simulink model "COMPONENT_MDL_Lag_QUAD_and_PEND_with_spin_rotors"  (R2021b)
(part 5 of 10)

    mt33 = [et183+et184+et185+et186+et187+et188+et189+et190+et191+et192+et193+et194+et195+et196+et197+et198+et199+et200+et201+et202+et203+et204+et205+et206+et207+et208+et209+et210+et211+et212+et213+et214+et215+et216+et217+et218+et219+et220+et221+et222+et223+et224,et149+et150+et151+et152+et153+et154+et155+et156+et157+et158+et159+et160+et161+et162+et163+et164+et165+et166+et167+et168+et169+et170+et171+et172+et173+et174+et175+et176+et177+et178+et179+et180+et181+et182,et124+et125+et126+et127+et128+et129+et130+et131+et132+et133+et134+et135+et136+et137+et138+et139+et140+et141+et142+et143+et144+et145+et146+et147+et148,et120+et121+et122+et123,et116+et117+et118+et119,0.0,et96+et97+et98+et99+et100+et101+et102+et103+et104+et105+et106+et107+et108+et109+et110+et111+et112+et113+et114+et115,et77+et78+et79+et80+et81+et82+et83+et84+et85+et86+et87+et88+et89+et90+et91+et92+et93+et94+et95,et59+et60+et61+et62+et63+et64+et65+et66+et67+et68+et69+et70+et71+et72+et73+et74+et75+et76];
    mt34 = [et272+et273+et274+et275+et276+et277+et278+et279+et280+et281+et282+et283+et284+et285+et286+et287+et288+et289+et290+et291+et292+et293+et294+et295+et296+et297+et298+et299,et260+et261+et262+et263+et264+et265+et266+et267+et268+et269+et270+et271,et250+et251+et252+et253+et254+et255+et256+et257+et258+et259,cos(THE_Phi).*(et248+et249).*(-1.0./2.0),sin(THE_Phi).*(et246+et247).*(-1.0./2.0),et244+et245,et237+et238+et239+et240+et241+et242+et243,et231+et232+et233+et234+et235+et236,et225+et226+et227+et228+et229+et230,et321+et322+et323+et324+et325+et326+et327+et328+et329+et330+et331,et313+et314+et315+et316+et317+et318+et319+et320,et310+et311+et312,et308+et309,et306+et307];
    mt35 = [cos(THE_Theta).*(THE_Psi_D.*Tv_Z_pend.*m_pend.*cos(THE_Psi).*2.0+THE_Psi_D.*cg_to_mot_H.*mprop.*cos(THE_Psi).*8.0+Lz_pend.*THE_Psi_D.*m_pend.*cos(THE_Psi).*cos(THE_Psi_pend).*cos(THE_Theta_pend)+Lz_pend.*THE_Psi_pend_D.*m_pend.*cos(THE_Psi).*cos(THE_Phi_pend).*cos(THE_Psi_pend).*2.0-Lz_pend.*THE_Psi_D.*m_pend.*cos(THE_Phi_pend).*sin(THE_Psi).*sin(THE_Psi_pend)-Lz_pend.*THE_Phi_pend_D.*m_pend.*cos(THE_Psi).*sin(THE_Phi_pend).*sin(THE_Psi_pend).*2.0-Lz_pend.*THE_Psi_pend_D.*m_pend.*cos(THE_Theta_pend).*sin(THE_Psi).*sin(THE_Psi_pend).*2.0-Lz_pend.*THE_Theta_pend_D.*m_pend.*cos(THE_Psi_pend).*sin(THE_Psi).*sin(THE_Theta_pend).*2.0-Lz_pend.*THE_Phi_pend_D.*m_pend.*cos(THE_Psi).*cos(THE_Phi_pend).*cos(THE_Psi_pend).*sin(THE_Theta_pend).*2.0-Lz_pend.*THE_Theta_pend_D.*m_pend.*cos(THE_Psi).*cos(THE_Psi_pend).*cos(THE_Theta_pend).*sin(THE_Phi_pend).*2.0+Lz_pend.*THE_Psi_D.*m_pend.*cos(THE_Psi_pend).*sin(THE_Psi).*sin(THE_Phi_pend).*sin(THE_Theta_pend)+Lz_pend.*THE_Psi_pend_D.*m_pend.*cos(THE_Psi).*sin(THE_Phi_pend).*sin(THE_Psi_pend).*sin(THE_Theta_pend).*2.0).*(-1.0./2.0),(m_pend.*(et304+et305))./1.2e+1,et302+et303,m_pend.*(et300+et301).*(-1.0./1.2e+1),0.0,0.0,0.0,0.0,0.0,0.0,0.0,0.0,0.0,0.0,0.0,0.0,0.0,0.0,0.0,0.0,0.0,0.0,0.0,0.0,0.0,0.0,0.0,0.0,0.0,0.0,0.0,et342+et343+et344+et345+et346];
    mt36 = [et339+et340+et341,et337+et338,et335.*et336,et332.*et333.*et334,(Lz_pend.*m_pend.*(THE_Phi_pend_D.*sin(THE_Theta).*sin(THE_Phi_pend).*sin(THE_Psi_pend)-THE_Psi_pend_D.*cos(THE_Phi_pend).*cos(THE_Psi_pend).*sin(THE_Theta).*2.0+THE_Phi_pend_D.*cos(THE_Theta).*cos(THE_Phi_pend).*sin(THE_Psi).*sin(THE_Psi_pend)+THE_Psi_pend_D.*cos(THE_Theta).*cos(THE_Psi_pend).*sin(THE_Psi).*sin(THE_Phi_pend).*2.0+THE_Phi_pend_D.*cos(THE_Phi_pend).*cos(THE_Psi_pend).*sin(THE_Theta).*sin(THE_Theta_pend)+THE_Theta_pend_D.*cos(THE_Psi_pend).*cos(THE_Theta_pend).*sin(THE_Theta).*sin(THE_Phi_pend).*2.0-THE_Psi_pend_D.*sin(THE_Theta).*sin(THE_Phi_pend).*sin(THE_Psi_pend).*sin(THE_Theta_pend).*2.0+THE_Theta_pend_D.*cos(THE_Theta).*cos(THE_Phi_pend).*cos(THE_Psi_pend).*cos(THE_Theta_pend).*sin(THE_Psi).*2.0-THE_Phi_pend_D.*cos(THE_Theta).*cos(THE_Psi_pend).*sin(THE_Psi).*sin(THE_Phi_pend).*sin(THE_Theta_pend)-THE_Psi_pend_D.*cos(THE_Theta).*cos(THE_Phi_pend).*sin(THE_Psi).*sin(THE_Psi_pend).*sin(THE_Theta_pend).*2.0))./2.0];
    mt37 = [m_pend.*cos(THE_Theta_pend).*(Lx_pend.^2.*THE_Theta_pend_D.*sin(THE_Theta_pend)-Ly_pend.^2.*THE_Theta_pend_D.*sin(THE_Theta_pend)+Ly_pend.^2.*THE_Theta_pend_D.*cos(THE_Psi_pend).^2.*sin(THE_Theta_pend)-Lz_pend.^2.*THE_Theta_pend_D.*cos(THE_Psi_pend).^2.*sin(THE_Theta_pend).*4.0+Ly_pend.^2.*THE_Psi_pend_D.*cos(THE_Psi_pend).*cos(THE_Theta_pend).*sin(THE_Psi_pend)-Lz_pend.^2.*THE_Psi_pend_D.*cos(THE_Psi_pend).*cos(THE_Theta_pend).*sin(THE_Psi_pend).*4.0).*(-1.0./6.0),(m_pend.*cos(THE_Theta_pend).*(Ly_pend.^2.*THE_Psi_pend_D.*2.0+Lx_pend.^2.*THE_Phi_pend_D.*sin(THE_Theta_pend)-Ly_pend.^2.*THE_Phi_pend_D.*sin(THE_Theta_pend)-Ly_pend.^2.*THE_Psi_pend_D.*cos(THE_Psi_pend).^2.*2.0+Lz_pend.^2.*THE_Psi_pend_D.*cos(THE_Psi_pend).^2.*8.0+Ly_pend.^2.*THE_Phi_pend_D.*cos(THE_Psi_pend).^2.*sin(THE_Theta_pend)-Lz_pend.^2.*THE_Phi_pend_D.*cos(THE_Psi_pend).^2.*sin(THE_Theta_pend).*4.0))./1.2e+1];
    mt38 = [m_pend.*cos(THE_Theta_pend).*(Ly_pend.^2.*THE_Theta_pend_D.*2.0-Ly_pend.^2.*THE_Theta_pend_D.*cos(THE_Psi_pend).^2.*2.0+Lz_pend.^2.*THE_Theta_pend_D.*cos(THE_Psi_pend).^2.*8.0-Ly_pend.^2.*THE_Phi_pend_D.*cos(THE_Psi_pend).*cos(THE_Theta_pend).*sin(THE_Psi_pend)+Lz_pend.^2.*THE_Phi_pend_D.*cos(THE_Psi_pend).*cos(THE_Theta_pend).*sin(THE_Psi_pend).*4.0).*(-1.0./1.2e+1),et349+et350+et351,et347+et348];
    mt39 = [Lz_pend.^2.*THE_Psi_pend_D.*m_pend.*cos(THE_Phi_pend).*sin(THE_Theta_pend).*(-2.0./3.0)-(Ly_pend.^2.*THE_Psi_pend_D.*m_pend.*cos(THE_Psi_pend).*sin(THE_Phi_pend).*sin(THE_Psi_pend))./6.0+Lz_pend.^2.*THE_Psi_pend_D.*m_pend.*cos(THE_Psi_pend).*sin(THE_Phi_pend).*sin(THE_Psi_pend).*(2.0./3.0)-(Ly_pend.^2.*THE_Psi_pend_D.*m_pend.*cos(THE_Phi_pend).*cos(THE_Psi_pend).^2.*sin(THE_Theta_pend))./6.0+Lz_pend.^2.*THE_Psi_pend_D.*m_pend.*cos(THE_Phi_pend).*cos(THE_Psi_pend).^2.*sin(THE_Theta_pend).*(2.0./3.0)+Lz_pend.*THE_Psi_pend_D.*Tv_Z_pend.*m_pend.*cos(THE_Theta_pend).*sin(THE_Phi_pend).*sin(THE_Psi_pend)+(Lz_pend.*THE_Theta_pend_D.*Tv_Z_pend.*m_pend.*cos(THE_Psi_pend).*sin(THE_Phi_pend).*sin(THE_Theta_pend))./2.0-(Ly_pend.^2.*THE_Theta_pend_D.*m_pend.*cos(THE_Phi_pend).*cos(THE_Psi_pend).*cos(THE_Theta_pend).*sin(THE_Psi_pend))./1.2e+1+(Lz_pend.^2.*THE_Theta_pend_D.*m_pend.*cos(THE_Phi_pend).*cos(THE_Psi_pend).*cos(THE_Theta_pend).*sin(THE_Psi_pend))./3.0];
    mt40 = [Lz_pend.*m_pend.*(THE_Theta_pend_D.*cos(THE_Psi_pend).*cos(THE_Theta_pend).*sin(THE_Phi).*sin(THE_Psi)-THE_Psi_pend_D.*sin(THE_Phi).*sin(THE_Psi).*sin(THE_Psi_pend).*sin(THE_Theta_pend).*2.0+THE_Theta_pend_D.*cos(THE_Phi).*cos(THE_Psi).*cos(THE_Psi_pend).*cos(THE_Theta_pend).*sin(THE_Theta)+THE_Psi_pend_D.*cos(THE_Phi).*cos(THE_Theta).*cos(THE_Phi_pend).*cos(THE_Theta_pend).*sin(THE_Psi_pend).*2.0+THE_Theta_pend_D.*cos(THE_Phi).*cos(THE_Theta).*cos(THE_Phi_pend).*cos(THE_Psi_pend).*sin(THE_Theta_pend)-THE_Psi_pend_D.*cos(THE_Phi).*cos(THE_Psi).*sin(THE_Theta).*sin(THE_Psi_pend).*sin(THE_Theta_pend).*2.0-THE_Psi_pend_D.*cos(THE_Psi).*cos(THE_Theta_pend).*sin(THE_Phi).*sin(THE_Phi_pend).*sin(THE_Psi_pend).*2.0-THE_Theta_pend_D.*cos(THE_Psi).*cos(THE_Psi_pend).*sin(THE_Phi).*sin(THE_Phi_pend).*sin(THE_Theta_pend)+THE_Psi_pend_D.*cos(THE_Phi).*cos(THE_Theta_pend).*sin(THE_Psi).*sin(THE_Theta).*sin(THE_Phi_pend).*sin(THE_Psi_pend).*2.0+THE_Theta_pend_D.*cos(THE_Phi).*cos(THE_Psi_pend).*sin(THE_Psi).*sin(THE_Theta).*sin(THE_Phi_pend).*sin(THE_Theta_pend)).*(-1.0./2.0)];
    mt41 = [Lz_pend.*m_pend.*(-THE_Theta_pend_D.*cos(THE_Phi).*cos(THE_Psi_pend).*cos(THE_Theta_pend).*sin(THE_Psi)+THE_Psi_pend_D.*cos(THE_Phi).*sin(THE_Psi).*sin(THE_Psi_pend).*sin(THE_Theta_pend).*2.0+THE_Theta_pend_D.*cos(THE_Psi).*cos(THE_Psi_pend).*cos(THE_Theta_pend).*sin(THE_Phi).*sin(THE_Theta)+THE_Psi_pend_D.*cos(THE_Phi).*cos(THE_Psi).*cos(THE_Theta_pend).*sin(THE_Phi_pend).*sin(THE_Psi_pend).*2.0+THE_Psi_pend_D.*cos(THE_Theta).*cos(THE_Phi_pend).*cos(THE_Theta_pend).*sin(THE_Phi).*sin(THE_Psi_pend).*2.0+THE_Theta_pend_D.*cos(THE_Phi).*cos(THE_Psi).*cos(THE_Psi_pend).*sin(THE_Phi_pend).*sin(THE_Theta_pend)+THE_Theta_pend_D.*cos(THE_Theta).*cos(THE_Phi_pend).*cos(THE_Psi_pend).*sin(THE_Phi).*sin(THE_Theta_pend)-THE_Psi_pend_D.*cos(THE_Psi).*sin(THE_Phi).*sin(THE_Theta).*sin(THE_Psi_pend).*sin(THE_Theta_pend).*2.0+THE_Psi_pend_D.*cos(THE_Theta_pend).*sin(THE_Phi).*sin(THE_Psi).*sin(THE_Theta).*sin(THE_Phi_pend).*sin(THE_Psi_pend).*2.0+THE_Theta_pend_D.*cos(THE_Psi_pend).*sin(THE_Phi).*sin(THE_Psi).*sin(THE_Theta).*sin(THE_Phi_pend).*sin(THE_Theta_pend)).*(-1.0./2.0)];
    mt42 = [Lz_pend.*m_pend.*(THE_Theta_pend_D.*cos(THE_Psi).*cos(THE_Theta).*cos(THE_Psi_pend).*cos(THE_Theta_pend)-THE_Psi_pend_D.*cos(THE_Psi).*cos(THE_Theta).*sin(THE_Psi_pend).*sin(THE_Theta_pend).*2.0-THE_Psi_pend_D.*cos(THE_Phi_pend).*cos(THE_Theta_pend).*sin(THE_Theta).*sin(THE_Psi_pend).*2.0-THE_Theta_pend_D.*cos(THE_Phi_pend).*cos(THE_Psi_pend).*sin(THE_Theta).*sin(THE_Theta_pend)+THE_Psi_pend_D.*cos(THE_Theta).*cos(THE_Theta_pend).*sin(THE_Psi).*sin(THE_Phi_pend).*sin(THE_Psi_pend).*2.0+THE_Theta_pend_D.*cos(THE_Theta).*cos(THE_Psi_pend).*sin(THE_Psi).*sin(THE_Phi_pend).*sin(THE_Theta_pend)).*(-1.0./2.0),m_pend.*(Lz_pend.^2.*THE_Psi_pend_D.*cos(THE_Theta_pend).*8.0+Ly_pend.^2.*THE_Psi_pend_D.*cos(THE_Psi_pend).^2.*cos(THE_Theta_pend).*2.0-Lz_pend.^2.*THE_Psi_pend_D.*cos(THE_Psi_pend).^2.*cos(THE_Theta_pend).*8.0-Ly_pend.^2.*THE_Theta_pend_D.*cos(THE_Psi_pend).*sin(THE_Psi_pend).*sin(THE_Theta_pend)+Lz_pend.^2.*THE_Theta_pend_D.*cos(THE_Psi_pend).*sin(THE_Psi_pend).*sin(THE_Theta_pend).*4.0).*(-1.0./1.2e+1),(THE_Psi_pend_D.*m_pend.*sin(THE_Psi_pend.*2.0).*(Ly_pend.^2-Lz_pend.^2.*4.0))./1.2e+1,THE_Theta_pend_D.*m_pend.*sin(THE_Psi_pend.*2.0).*(Ly_pend.^2-Lz_pend.^2.*4.0).*(-1.0./2.4e+1)];
    mt43 = [Lz_pend.*THE_Psi_pend_D.*Tv_Z_pend.*m_pend.*(-cos(THE_Phi_pend).*sin(THE_Theta).*sin(THE_Psi_pend)+cos(THE_Theta).*sin(THE_Psi).*sin(THE_Phi_pend).*sin(THE_Psi_pend)+cos(THE_Psi_pend).*sin(THE_Theta).*sin(THE_Phi_pend).*sin(THE_Theta_pend)+cos(THE_Theta).*cos(THE_Phi_pend).*cos(THE_Psi_pend).*sin(THE_Psi).*sin(THE_Theta_pend)).*(-1.0./2.0),Lz_pend.*THE_Psi_pend_D.*Tv_Z_pend.*m_pend.*cos(THE_Psi).*(sin(THE_Phi_pend).*sin(THE_Psi_pend)+cos(THE_Phi_pend).*cos(THE_Psi_pend).*sin(THE_Theta_pend)).*(-1.0./2.0),Lz_pend.*THE_Psi_pend_D.*Tv_Z_pend.*m_pend.*(cos(THE_Phi_pend).*sin(THE_Psi_pend)-cos(THE_Psi_pend).*sin(THE_Phi_pend).*sin(THE_Theta_pend)).*(-1.0./2.0),Lz_pend.*THE_Psi_pend_D.*m_pend.*(cos(THE_Psi).*cos(THE_Phi_pend).*sin(THE_Phi).*sin(THE_Psi_pend)+cos(THE_Phi).*cos(THE_Theta).*sin(THE_Phi_pend).*sin(THE_Psi_pend)+cos(THE_Psi_pend).*cos(THE_Theta_pend).*sin(THE_Phi).*sin(THE_Psi)+cos(THE_Phi).*cos(THE_Psi).*cos(THE_Psi_pend).*cos(THE_Theta_pend).*sin(THE_Theta)+cos(THE_Phi).*cos(THE_Theta).*cos(THE_Phi_pend).*cos(THE_Psi_pend).*sin(THE_Theta_pend)-cos(THE_Phi).*cos(THE_Phi_pend).*sin(THE_Psi).*sin(THE_Theta).*sin(THE_Psi_pend)-cos(THE_Psi).*cos(THE_Psi_pend).*sin(THE_Phi).*sin(THE_Phi_pend).*sin(THE_Theta_pend)+cos(THE_Phi).*cos(THE_Psi_pend).*sin(THE_Psi).*sin(THE_Theta).*sin(THE_Phi_pend).*sin(THE_Theta_pend)).*(-1.0./2.0)];
    mt44 = [Lz_pend.*THE_Psi_pend_D.*m_pend.*(-cos(THE_Phi).*cos(THE_Psi).*cos(THE_Phi_pend).*sin(THE_Psi_pend)-cos(THE_Phi).*cos(THE_Psi_pend).*cos(THE_Theta_pend).*sin(THE_Psi)+cos(THE_Theta).*sin(THE_Phi).*sin(THE_Phi_pend).*sin(THE_Psi_pend)+cos(THE_Psi).*cos(THE_Psi_pend).*cos(THE_Theta_pend).*sin(THE_Phi).*sin(THE_Theta)+cos(THE_Phi).*cos(THE_Psi).*cos(THE_Psi_pend).*sin(THE_Phi_pend).*sin(THE_Theta_pend)+cos(THE_Theta).*cos(THE_Phi_pend).*cos(THE_Psi_pend).*sin(THE_Phi).*sin(THE_Theta_pend)-cos(THE_Phi_pend).*sin(THE_Phi).*sin(THE_Psi).*sin(THE_Theta).*sin(THE_Psi_pend)+cos(THE_Psi_pend).*sin(THE_Phi).*sin(THE_Psi).*sin(THE_Theta).*sin(THE_Phi_pend).*sin(THE_Theta_pend)).*(-1.0./2.0),(Lz_pend.*THE_Psi_pend_D.*m_pend.*(sin(THE_Theta).*sin(THE_Phi_pend).*sin(THE_Psi_pend)-cos(THE_Psi).*cos(THE_Theta).*cos(THE_Psi_pend).*cos(THE_Theta_pend)+cos(THE_Theta).*cos(THE_Phi_pend).*sin(THE_Psi).*sin(THE_Psi_pend)+cos(THE_Phi_pend).*cos(THE_Psi_pend).*sin(THE_Theta).*sin(THE_Theta_pend)-cos(THE_Theta).*cos(THE_Psi_pend).*sin(THE_Psi).*sin(THE_Phi_pend).*sin(THE_Theta_pend)))./2.0,0.0,0.0,0.0];
    C = reshape([mt33,mt34,mt35,mt36,mt37,mt38,mt39,mt40,mt41,mt42,mt43,mt44],9,9);
end
if nargout > 2
    K = reshape([0.0,0.0,0.0,0.0,0.0,0.0,0.0,0.0,0.0,0.0,0.0,0.0,0.0,0.0,0.0,0.0,0.0,0.0,0.0,0.0,0.0,0.0,0.0,0.0,0.0,0.0,0.0,0.0,0.0,0.0,0.0,0.0,0.0,0.0,0.0,0.0,0.0,0.0,0.0,0.0,0.0,0.0,0.0,0.0,0.0,0.0,0.0,0.0,0.0,0.0,0.0,0.0,0.0,0.0,0.0,0.0,0.0,0.0,0.0,0.0,0.0,0.0,0.0,0.0,0.0,0.0,0.0,0.0,0.0,0.0,0.0,0.0,0.0,0.0,0.0,0.0,0.0,0.0,0.0,0.0,0.0],[9,9]);
end
if nargout > 3
    mt45 = [0.0,-Tv_Z_pend.*g.*m_pend.*cos(THE_Psi).*sin(THE_Theta)-cg_to_mot_H.*g.*mprop.*cos(THE_Psi).*sin(THE_Theta).*4.0-(Lz_pend.*g.*m_pend.*cos(THE_Theta).*sin(THE_Phi_pend).*sin(THE_Psi_pend))./2.0-(Lz_pend.*g.*m_pend.*cos(THE_Psi).*cos(THE_Psi_pend).*cos(THE_Theta_pend).*sin(THE_Theta))./2.0-(Lz_pend.*g.*m_pend.*cos(THE_Theta).*cos(THE_Phi_pend).*cos(THE_Psi_pend).*sin(THE_Theta_pend))./2.0+(Lz_pend.*g.*m_pend.*cos(THE_Phi_pend).*sin(THE_Psi).*sin(THE_Theta).*sin(THE_Psi_pend))./2.0-(Lz_pend.*g.*m_pend.*cos(THE_Psi_pend).*sin(THE_Psi).*sin(THE_Theta).*sin(THE_Phi_pend).*sin(THE_Theta_pend))./2.0,g.*cos(THE_Theta).*(Tv_Z_pend.*m_pend.*sin(THE_Psi).*2.0+cg_to_mot_H.*mprop.*sin(THE_Psi).*8.0+Lz_pend.*m_pend.*cos(THE_Psi).*cos(THE_Phi_pend).*sin(THE_Psi_pend)+Lz_pend.*m_pend.*cos(THE_Psi_pend).*cos(THE_Theta_pend).*sin(THE_Psi)-Lz_pend.*m_pend.*cos(THE_Psi).*cos(THE_Psi_pend).*sin(THE_Phi_pend).*sin(THE_Theta_pend)).*(-1.0./2.0),0.0,0.0,g.*(m+m_pend+mprop.*4.0)];
    mt46 = [(Lz_pend.*g.*m_pend.*(-cos(THE_Phi_pend).*sin(THE_Theta).*sin(THE_Psi_pend)+cos(THE_Theta).*sin(THE_Psi).*sin(THE_Phi_pend).*sin(THE_Psi_pend)+cos(THE_Psi_pend).*sin(THE_Theta).*sin(THE_Phi_pend).*sin(THE_Theta_pend)+cos(THE_Theta).*cos(THE_Phi_pend).*cos(THE_Psi_pend).*sin(THE_Psi).*sin(THE_Theta_pend)))./2.0,Lz_pend.*g.*m_pend.*cos(THE_Psi_pend).*(cos(THE_Psi).*cos(THE_Theta).*sin(THE_Theta_pend)+cos(THE_Phi_pend).*cos(THE_Theta_pend).*sin(THE_Theta)-cos(THE_Theta).*cos(THE_Theta_pend).*sin(THE_Psi).*sin(THE_Phi_pend)).*(-1.0./2.0),Lz_pend.*g.*m_pend.*(cos(THE_Psi_pend).*sin(THE_Theta).*sin(THE_Phi_pend)+cos(THE_Theta).*cos(THE_Phi_pend).*cos(THE_Psi_pend).*sin(THE_Psi)+cos(THE_Psi).*cos(THE_Theta).*cos(THE_Theta_pend).*sin(THE_Psi_pend)-cos(THE_Phi_pend).*sin(THE_Theta).*sin(THE_Psi_pend).*sin(THE_Theta_pend)+cos(THE_Theta).*sin(THE_Psi).*sin(THE_Phi_pend).*sin(THE_Psi_pend).*sin(THE_Theta_pend)).*(-1.0./2.0)];
    G = reshape([mt45,mt46],9,1);
end
if nargout > 4
    Q = [Mbz_1.*cos(THE_Psi).*cos(THE_Theta)+Mbz_2.*cos(THE_Psi).*cos(THE_Theta)+Mbz_3.*cos(THE_Psi).*cos(THE_Theta)+Mbz_4.*cos(THE_Psi).*cos(THE_Theta)-Tbz_2.*cg_to_mot_L.*sin(THE_Theta)+Tbz_4.*cg_to_mot_L.*sin(THE_Theta)-Tbz_1.*cg_to_mot_L.*cos(THE_Theta).*sin(THE_Psi)+Tbz_3.*cg_to_mot_L.*cos(THE_Theta).*sin(THE_Psi);-Mbz_1.*sin(THE_Psi)-Mbz_2.*sin(THE_Psi)-Mbz_3.*sin(THE_Psi)-Mbz_4.*sin(THE_Psi)-Tbz_1.*cg_to_mot_L.*cos(THE_Psi)+Tbz_3.*cg_to_mot_L.*cos(THE_Psi);cg_to_mot_L.*(Tbz_2-Tbz_4);(sin(THE_Phi).*sin(THE_Psi)+cos(THE_Phi).*cos(THE_Psi).*sin(THE_Theta)).*(Tbz_1+Tbz_2+Tbz_3+Tbz_4);-(cos(THE_Phi).*sin(THE_Psi)-cos(THE_Psi).*sin(THE_Phi).*sin(THE_Theta)).*(Tbz_1+Tbz_2+Tbz_3+Tbz_4);cos(THE_Psi).*cos(THE_Theta).*(Tbz_1+Tbz_2+Tbz_3+Tbz_4);0.0;0.0;0.0];
end
